simulink model "SimulacionT1P2"  (R2022b)
settings: Solver=VariableStepAuto  StartTime=0.0  StopTime=10.0  RelTol=1e-3
settings Model: Creator=David  LastModifiedBy=David

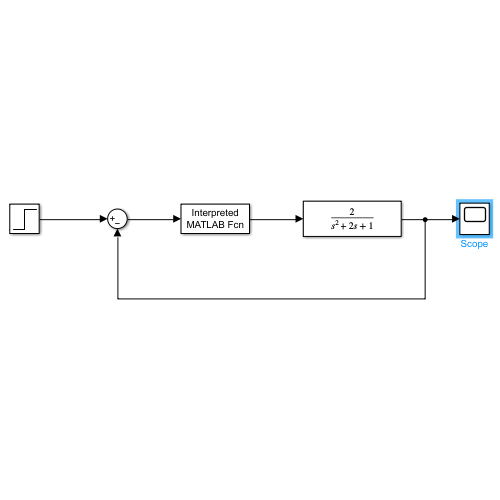
[thumbnail: Simulink's stored preview of the top-level diagram]
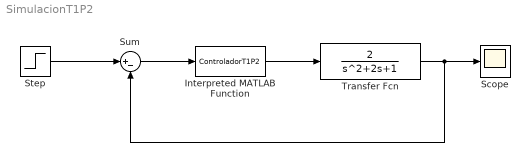
== system SimulacionT1P2 ==
  Interpreted MATLAB Function : MATLABFcn  MATLABFcn=ControladorT1P2
  Scope : Scope
  Step : Step  SampleTime=0
  Sum : Sum  Inputs=|+-
  Transfer Fcn : TransferFcn  Numerator=[2]
  wires:
  Step/1 -> Sum/1
  Sum/1 -> Interpreted MATLAB Function/1
  Interpreted MATLAB Function/1 -> Transfer Fcn/1
  Transfer Fcn/1 -> Sum/2, Scope/1
